simulink model "Tous_le_systeme_2020"  (R2020b)
settings: Solver=FixedStepAuto  StartTime=0.0  StopTime=0.3  FixedStep=1e-6  RelTol=1e-3
undefined symbols (not defined in the file or in its folder): FC, FuelCellLoadFcn, gcbh, ln, sps_rtmsupport, Ts
libraries: simulink x14, powerlib x13, powerlib_meascontrol x3, powerlib_extras x2, pid_lib x1
settings Model: Creator=Abdelhak_Samir  LastModifiedBy=Abdelhak_Samir
settings SolverCC: ZeroCrossAlgorithm=Adaptive
settings DebuggingCC: IgnoredZcDiagnostic=none  UnconnectedInputMsg=none  UnconnectedOutputMsg=none  UnconnectedLineMsg=none
settings ModelReferenceCC: EnableRefExpFcnMdlSchedulingChecks=off

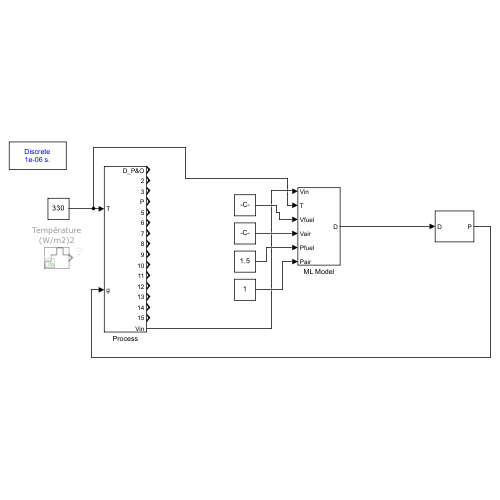
[thumbnail: Simulink's stored preview of the top-level diagram]
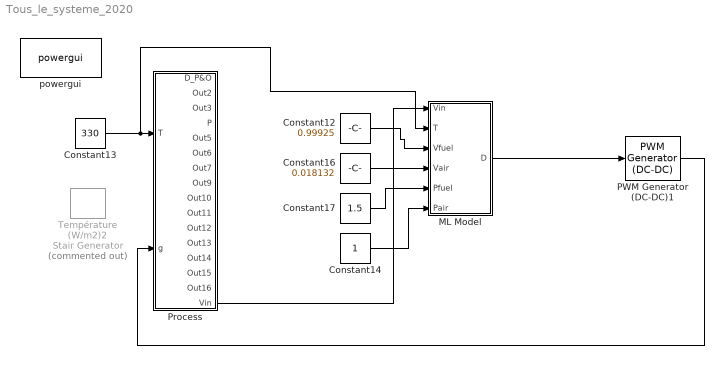
== system Tous_le_systeme_2020 ==
  Constant12 : Constant  Value=0.99925
  Constant13 : Constant  Value=330
  Constant14 : Constant
  Constant16 : Constant  Value=0.018132
  Constant17 : Constant  Value=1.5
  ML Model : Subsystem
  PWM Generator (DC-DC)1 : powerlib_meascontrol/Pulse & Signal Generators/PWM Generator (DC-DC)  Fsw=1/(2e-5)  Ts=1e-6
  Process : Subsystem
  Température (W/m2)2 : powerlib_meascontrol/Pulse & Signal Generators/Stair Generator  Commented=on  t=[0, 0.2 , 0.4 , 0.6, 0.8,1]  e=[300,310,320,330,320,320]  Ts=0.00001
  powergui : powerlib/powergui  Priority=1  SimulationMode=Discrete  SampleTime=1e-6  frequency=60  Iterations=50  frequencyindice=0  Pbase=100e6  ErrMax=1e-4  UnitsV=kV  UnitsW=MW  buscounter=0  FunctionMessages=off  echomessages=off  EnableUseOfTLC=off  CurrentSourceSwitches=off  DisableSnubberDevices=off  DisableRonSwitches=off  DisableVfSwitches=off  DisplayEquations=off  AutomaticDiscreteSolvers=off  SolverType=Tustin/Backward Euler (TBE)  Interpol=off  ExternalGateDelay=off  methode=off  Ts=100  x0status=blocks  SPID=on  SwTol=0  HookPort=off  NonlinearTolerance=1e-4  nMaxIteration=100  ContinueOnMaxIteration=off  RestoreLinks=warning  ResistiveCurrentMeasurement=off  Frange=[0:2:500]  Ylog=off  Xlog=on  ShowGrid=off  save=off  variable=ZData  structure=0  ZoomFFT=off  StartTime=0.0  cycles=1  DisplayStyle=1  fundamental=60  FreqAxis=off  MaxFrequency=1000  frequencyindicesteady=1  RmsSteady=1  display=off
  wires:
  Constant17/1 -> ML Model/5(Pfuel)
  Constant14/1 -> ML Model/6(Pair)
  Constant12/1 -> ML Model/3(Vfuel)
  Constant16/1 -> ML Model/4(Vair)
  Constant13/1 -> ML Model/2(T), Process/1(T)
  Process/16(Vin) -> ML Model/1(Vin)
  ML Model/1(D) -> PWM Generator (DC-DC)1/1
  PWM Generator (DC-DC)1/1 -> Process/2(g)

== system Tous_le_systeme_2020/ML Model ==
  Vin : Inport
  T : Inport  Port=2
  Vfuel : Inport  Port=3
  Vair : Inport  Port=4
  Pfuel : Inport  Port=5
  Pair : Inport  Port=6
  Display : Display
  MATLAB Function1 : MATLAB Function  TreatAsAtomicUnit=on
  MATLAB Function2 : MATLAB Function  Commented=on  TreatAsAtomicUnit=on
  PID Controller : pid_lib/PID Controller  Controller=PID  Form=Parallel  TimeDomain=Discrete-time  UseExternalTs=off  SampleTime=-1  IntegratorMethod=Forward Euler  ControllerParametersSource=internal  P=-150  I=-0.5  D=0.01  N=0  UseFilter=on  TunerSelectOption=Transfer Function Based (PID Tuner App)  InitialConditionSource=internal  InitialConditionForIntegrator=0  InitialConditionForFilter=0  DifferentiatorICPrevScaledInput=0  ExternalReset=none  TrackingMode=off  Kt=1  LimitOutput=off  SatLimitsSource=internal  UpperSaturationLimit=inf  LowerSaturationLimit=-inf  LinearizeAsGain=on  AntiWindupMode=none  Kb=1  POutMin=[]  POutMax=[]  IOutMin=[]  IOutMax=[]  DOutMin=[]  DOutMax=[]  NOutMin=[]  NOutMax=[]  SumOutMin=[]  SumOutMax=[]  SaturationOutMin=[]  SaturationOutMax=[]  PParamMin=[]  PParamMax=[]  IParamMin=[]  IParamMax=[]  DParamMin=[]  DParamMax=[]  NParamMin=[]  NParamMax=[]  KbParamMin=[]  KbParamMax=[]  KtParamMin=[]  KtParamMax=[]  KbOutMin=[]  KbOutMax=[]  KtOutMin=[]  KtOutMax=[]  IntegratorOutMin=[]  IntegratorOutMax=[]  FilterOutMin=[]  FilterOutMax=[]  SumI1OutMin=[]  SumI1OutMax=[]  SumI2OutMin=[]  SumI2OutMax=[]  SumI3OutMin=[]  SumI3OutMax=[]  SumI4OutMin=[]  SumI4OutMax=[]  SumDOutMin=[]  SumDOutMax=[]  DifferentiatorOutMin=[]  DifferentiatorOutMax=[]  FilterDiffOutCoefMin=[]  FilterDiffOutCoefMax=[]  ReciprocalOutMin=[]  ReciprocalOutMax=[]  SumDenOutMin=[]  SumDenOutMax=[]  SumNumOutMin=[]  SumNumOutMax=[]  DivideOutMin=[]  DivideOutMax=[]  UdiffTsProdOutMin=[]  UdiffTsProdOutMax=[]  NTsProdOutMin=[]  NTsProdOutMax=[]  UintegralTsProdOutMin=[]  UintegralTsProdOutMax=[]  UngainTsProdOutMin=[]  UngainTsProdOutMax=[]  IntegratorContinuousStateAttributes=''  IntegratorStateMustResolveToSignalObject=off  IntegratorRTWStateStorageClass=Auto  FilterContinuousStateAttributes=''  FilterStateMustResolveToSignalObject=off  FilterRTWStateStorageClass=Auto  ParallelPVariant=InternalParameters  IdealPVariant=Disabled  IVariant=InternalParameters  DVariant=InternalParameters  IntegratorVariant=Discrete  SatVariant=Disabled  AWVariant=Passthrough  PCopyVariant=Disabled  TRVariant=Disabled  FdbkBlocksVariant=Forward  IdealPFdbkVariant=Disabled  SatFdbkVariant=Disabled  DerivativeFilterVariant=ForwardEulerFilter  NVariant=InternalParameters  NCopyVariant=Disabled  FilterICVariant=InternalICsFilter  IntegratorICVariant=InternalICs  ExternalResetVariant=Disabled  TRSumVariant=Passthrough  SumFdbkVariant=Disabled  SumVariant=Sum_PID  TsampFilterVariant=InternalTs  TsampNgainVariant=Passthrough  TsampIntegralVariant=Disabled_SignalSpec  ExternalSaturationOutDataTypeStr=Inherit: Same as second input
  Saturation1 : Saturate  UpperLimit=0.9  LowerLimit=0.1
  Sum2 : Sum  Inputs=|+-
  D : Outport
  wires:
  Vair/1 -> MATLAB Function1/5(Vair)
  Pfuel/1 -> MATLAB Function1/2(Pfuel)
  T/1 -> MATLAB Function1/1(T)
  Vfuel/1 -> MATLAB Function1/4(Vfuel)
  Pair/1 -> MATLAB Function1/3(Pair)
  Sum2/1 -> PID Controller/1  "Vref-Vin"
  PID Controller/1 -> Saturation1/1
  Vin/1 -> Sum2/2
  Saturation1/1 -> D/1
  MATLAB Function1/1(vmpp) -> Sum2/1, Display/1  "Vref"

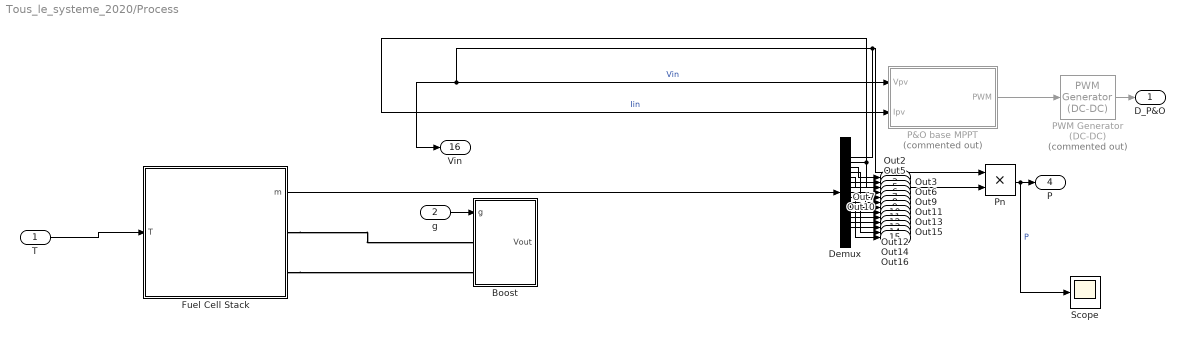
== system Tous_le_systeme_2020/Process ==
  T : Inport
  g : Inport  Port=2
  Boost : Subsystem
  Demux : Demux  Outputs=15
      settings: DisplayOption=none
  Fuel Cell Stack : Subsystem  AncestorBlock=sps_lib/Sources/Fuel Cell Stack  DialogController=POWERSYS.PowerSysDialog  LoadFcn=sps_rtmsupport('LoadFcn',gcbh);FuelCellLoadFcn(gcb)  StartFcn=sps_rtmsupport('StartFcn',gcbh);  StopFcn=sps_rtmsupport('StopFcn',gcbh);  mask(Fuel Cell Stack){PresetModel=PEMFC - 1.26 kW - 24 Vdc, FcType=0, Detailed=Detailed, Eoc=[42,35], NomVI=[52,24.23], EndVI=[100,20], Nc=42, n=46, TOp=55, AirFr=2400, SuppPress=[1.5,1], Comp=[99.95,21,1], SignX=off, SignY=off, FlowRateH2=off, FlowRateAir=off, SystemTemp=on, SystemPH2=off, SystemPAir=off, FCDyn=off, FC_tau=1e-6, Peak_O2=80, V_Under=10}
      mask prompts: PresetModel "Preset model:"; FcType "Fuel Cell type:"; Detailed "Model detail Level:"; Eoc "Voltage at 0A and 1A [V_0(V), V_1(V)]"; NomVI "Nominal operating point [Inom(A), Vnom(V)]"; EndVI "Maximum operating point [Iend(A), Vend(V)]"; Nc "Number of cells"; n "Nominal stack efficiency (%)"; TOp "Operating temperature (Celsius)"; AirFr "Nominal Air flow rate (lpm)"; SuppPress "Nominal supply pressure [Fuel (bar), Air (bar)]"; Comp "Nominal composition (%) [H2 O2 H2O(Air)]"; SignX "Fuel  composition [x_H2(%)]"; SignY "Oxidant composition [y_O2(%)]"; FlowRateH2 "Fuel flow rate [FuelFr(lpm)]"; FlowRateAir "Air flow rate [AirFr(lpm)]"; SystemTemp "System Temperature [T(Kelvin)]"; SystemPH2 "Fuel supply pressure [Pfuel(bar)]"; SystemPAir "Air supply pressure [PAir(bar)]"; FCDyn "Specify Fuel Cell Dynamics?"; FC_tau "Fuel Cell response time (sec)"; Peak_O2 "Peak O2 utilization (%)"; V_Under "Voltage undershoot (V) @ peak O2 utilization"
      mask help:
      | Implements a generic hydrogen fuel cell model which allows the simulation for the following types of cells:
      | - Proton Exchange Membrane Fuel Cell (PEMFC)
      | - Solid Oxide Fuel Cell (SOFC)
      | - Alkaline Fuel Cell (AFC)
      mask init:
      | block = gcb;
      | %% DO NOT CHANGE THIS ORDER
      | FuelCellCback(block,'Inputs')
      | [FC, WantBlockChoice, Ts] = FuelCellInit(block,Eoc,NomVI,EndVI,Nc,n,TOp,AirFr,SuppPress,Comp,FlowRateH2,FlowRateAir);
      | powericon('SetInternalModels','set',block,WantBlockChoice);
      settings: CopyFcn=sps_rtmsupport('CopyFcn',gcbh);  DeleteFcn=sps_rtmsupport('DeleteFcn',gcbh);  UndoDeleteFcn=sps_rtmsupport('UndoDeleteFcn',gcbh);  ModelCloseFcn=sps_rtmsupport('ModelCloseFcn',gcbh);  PreSaveFcn=sps_rtmsupport('PreSaveFcn',gcbh);  PostSaveFcn=sps_rtmsupport('PostSaveFcn',gcbh);  NameChangeFcn=sps_rtmsupport('NameChangeFcn',gcbh);  PreCopyFcn=sps_rtmsupport('PreCopyFcn',gcbh);  OpenFcn=sps_rtmsupport('OpenFcn',gcbh, [1 2 3 13 14 15 16 17 18 19 20]);  CloseFcn=sps_rtmsupport('CloseFcn',gcbh);  PreDeleteFcn=sps_rtmsupport('PreDeleteFcn',gcbh);
      mask Help: helpview(psbhelp)
      mask TypeOptions PresetModel: No (User-Defined) | PEMFC - 1.26 kW - 24 Vdc | PEMFC - 6 kW - 45 Vdc | PEMFC - 50 kW - 625 Vdc | AFC - 2.4 kW - 48 Vdc | SOFC - 3 kW - 100 Vdc | SOFC - 25 kW - 630 Vdc
      mask Callback PresetModel: FuelCellCback(gcb,'Preset')
      mask TypeOptions Detailed: Simplified | Detailed
      mask Callback Detailed: FuelCellCback(gcb,'Visibilities')
      mask Callback FlowRateAir: FuelCellCback(gcb,'Visibilities')
      mask Callback FCDyn: FuelCellCback(gcb,'Visibilities')
      mask DialogControl ParameterTabVar0 Prompt: Parameters
      mask DialogControl plot_graph Prompt: Plot V_I characteristic
      mask DialogControl plot_graph Callback: FuelCellCback(gcb,'PlotGraph');
      mask DialogControl ViewParam Prompt: View Cell parameters
      mask DialogControl ViewParam Callback: FuelCellCback(gcb,'ViewParam');
      mask DialogControl ParameterTabVar01 Prompt: Signal variation
      mask DialogControl ParameterTabVar012 Prompt: Fuel Cell Dynamics
  P&O base MPPT : Subsystem  Commented=on
  PWM Generator (DC-DC) : powerlib_meascontrol/Pulse & Signal Generators/PWM Generator (DC-DC)  Commented=on  Fsw=1/(2e-5)  Ts=1e-6
  Pn : Product
  Scope : Scope
  D_P&O : Outport
  Out2 : Outport  Port=2
  Out3 : Outport  Port=3
  P : Outport  Port=4
  Out5 : Outport  Port=5
  Out6 : Outport  Port=6
  Out7 : Outport  Port=7
  Out9 : Outport  Port=8
  Out10 : Outport  Port=9
  Out11 : Outport  Port=10
  Out12 : Outport  Port=11
  Out13 : Outport  Port=12
  Out14 : Outport  Port=13
  Out15 : Outport  Port=14
  Out16 : Outport  Port=15
  Vin : Outport  Port=16
  wires:
  PWM Generator (DC-DC)/1 -> D_P&O/1
  P&O base MPPT/1(PWM) -> PWM Generator (DC-DC)/1
  Demux/3 -> Out2/1
  Demux/12 -> Out13/1
  Demux/15 -> Out16/1
  Demux/11 -> Out12/1
  Fuel Cell Stack/1(m) -> Demux/1
  Demux/14 -> Out15/1
  Demux/1 -> Vin/1, P&O base MPPT/1(Vpv), Pn/1  "Vin"
  Demux/5 -> Out5/1
  Demux/2 -> Pn/2, P&O base MPPT/2(Ipv)  "Iin"
  T/1 -> Fuel Cell Stack/1(T)
  Demux/4 -> Out3/1
  Demux/9 -> Out10/1
  Demux/7 -> Out7/1
  Demux/6 -> Out6/1
  Demux/8 -> Out9/1
  Demux/10 -> Out11/1
  Demux/13 -> Out14/1
  Pn/1 -> Scope/1, P/1  "P"
  g/1 -> Boost/1(g)
  connections:
  Fuel Cell Stack/RConn1 -- Boost/LConn1
  Fuel Cell Stack/RConn2 -- Boost/LConn2

== system Tous_le_systeme_2020/Process/Boost ==
  note: Voltage Sensor
  note: Boost Convertor
  note: LOAD
  g : Inport
  Current Measurement : powerlib/Measurements/Current Measurement  PhasorSimulation=off  OutputType=Complex  PSBequivalent=0
  Diode : powerlib/Power Electronics/Diode  Ron=0.001  Lon=0  Vf=0.7  IC=0  UseSnubber=0  Rs=500  Cs=250e-9  Measurements=off
  Diode1 : powerlib/Power Electronics/Diode  Ron=0.001  Lon=0  Vf=0.7  IC=0  UseSnubber=0  Rs=500  Cs=250e-9  Measurements=off
  Divide : Product  Inputs=*/
  E1 : Product  Inputs=**
  Mosfet : powerlib/Power Electronics/Mosfet  Ron=0.1  Lon=0  Rd=0.01  Vfd=0.7  IC=0  Rs=1e5  Cs=10^-9  Measurements=off
  Scope : Scope  NumInputPorts=2
  Series RLC Branch : powerlib/Elements/Series RLC Branch  LConnTagsString=__new0  RConnTagsString=__new0  BranchType=L  Resistance=1  Inductance=1e-4  SetiL0=off  InitialCurrent=0  Capacitance=1e-6  Setx0=off  InitialVoltage=0  Measurements=None
  Series RLC Branch1 : powerlib/Elements/Series RLC Branch  LConnTagsString=__new0  RConnTagsString=__new0  BranchType=C  Resistance=1  Inductance=1e-4  SetiL0=off  InitialCurrent=0  Capacitance=4700e-6  Setx0=off  InitialVoltage=0  Measurements=None
  Series RLC Branch4 : powerlib/Elements/Series RLC Branch  LConnTagsString=__new0  RConnTagsString=__new0  BranchType=C  Resistance=1  Inductance=1e-4  SetiL0=off  InitialCurrent=0  Capacitance=4700e-5  Setx0=on  InitialVoltage=42  Measurements=None
  Series RLC Load1 : powerlib/Elements/Series RLC Load  LConnTagsString=a  RConnTagsString=__new0  NominalVoltage=50  NominalFrequency=500  ActivePower=33  InductivePower=0  CapacitivePower=0  Setx0=off  InitialVoltage=0  SetiL0=off  InitialCurrent=0  Measurements=None  LoadType=constant Z
  Voltage Measurement1 : powerlib/Measurements/Voltage Measurement  PhasorSimulation=off  OutputType=Complex  PSBequivalent=0
  a : PMIOPort  Side=Left
  Conn2 : PMIOPort  Port=2  Side=Left
  Vout : Outport
  wires:
  E1/1 -> Scope/1  "Pout"
  Voltage Measurement1/1 -> Vout/1, Divide/1, E1/2  "Vout"
  Current Measurement/1 -> Divide/2, E1/1  "Iout"
  g/1 -> Mosfet/1
  Divide/1 -> ?  "R"
  connections:
  Current Measurement/LConn1 -- Series RLC Branch1/LConn1 -- Diode/RConn1
  Voltage Measurement1/LConn2 -- Series RLC Branch1/RConn1 -- Series RLC Branch4/RConn1 -- Conn2/RConn1 -- Mosfet/RConn1 -- Series RLC Load1/RConn1
  Series RLC Load1/LConn1 -- Current Measurement/RConn1 -- Voltage Measurement1/LConn1
  a/RConn1 -- Diode1/LConn1
  Series RLC Branch/RConn1 -- Mosfet/LConn1 -- Diode/LConn1
  Diode1/RConn1 -- Series RLC Branch4/LConn1 -- Series RLC Branch/LConn1

== system Tous_le_systeme_2020/Process/Fuel Cell Stack ==
  T : Inport
  AirFr : Constant  Value=FC.Uf_O2
  Controlled Voltage Source1 : powerlib/Electrical Sources/Controlled Voltage Source  Initialize=on  Source_Type=AC  Amplitude=0  Phase=0  Frequency=0  Measurements=None
  Current Measurement1 : powerlib/Measurements/Current Measurement  PhasorSimulation=off  OutputType=Complex  PSBequivalent=0
  Diode1 : powerlib/Power Electronics/Diode  Ron=FC.Rohm  Lon=0  Vf=0  IC=0  UseSnubber=off  Rs=1e4  Cs=inf  Measurements=off
  FuelFr : Constant  Value=FC.Uf_H2
  Gain1 : Gain  Gain=0.01
  Gain3 : Gain  Gain=0.01
  Model : Subsystem  AncestorBlock=sps_lib/Sources/Fuel Cell Stack/Model  Variant=on  VariantControlMode=label  LabelModeActiveChoice=Discrete/Detailed
      settings: AttributesFormatString=%<BlockChoice>
  PAir : Constant  Value=FC.PAir
  Pfuel : Constant  Value=FC.Pf
  x_H2 : Constant  Value=FC.x*100
  y_O2 : Constant  Value=FC.y*100
  + : PMIOPort  Tag=PMCPort  Side=Right
  - : PMIOPort  Tag=PMCPort  Port=2  Side=Right
  m : Outport  VectorParamsAs1DForOutWhenUnconnected=off
  wires:
  PAir/1 -> Model/8(PAir)
  Pfuel/1 -> Model/7(Pf)
  T/1 -> Model/2(Op Temp)
  Model/1(Voltage) -> Controlled Voltage Source1/1
  Current Measurement1/1 -> Model/1(Current)
  Model/2(m) -> m/1
  FuelFr/1 -> Model/3(H2)
  x_H2/1 -> Gain1/1
  AirFr/1 -> Model/5(Air)
  y_O2/1 -> Gain3/1
  Gain1/1 -> Model/4(x_H2)
  Gain3/1 -> Model/6(y_O2)
  connections:
  Current Measurement1/LConn1 -- Controlled Voltage Source1/RConn1
  Current Measurement1/RConn1 -- Diode1/LConn1
  -/RConn1 -- Controlled Voltage Source1/LConn1
  Diode1/RConn1 -- +/RConn1

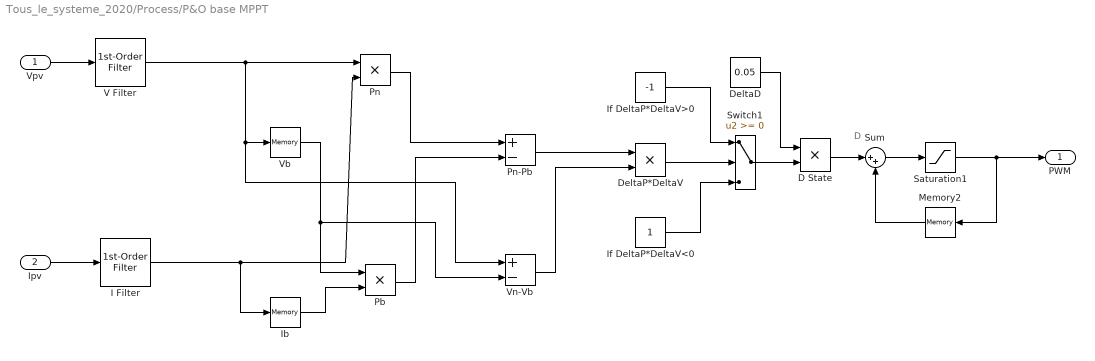
== system Tous_le_systeme_2020/Process/P&O base MPPT ==
  note: D
  Vpv : Inport
  Ipv : Inport  Port=2
  D State : Product  RndMeth=Zero
  DeltaD : Constant  Value=0.05
  DeltaP*DeltaV : Product  RndMeth=Zero
  I Filter : powerlib_extras/Control  Blocks/1st-Order  Filter  FilterType=Lowpass  Tc=1e-3  Initialize=off  Vac_Init=[0.8 -25 60]  Vdc_Init=-0.4  PlotResponse=off  param1=[1 500 1]
  Ib : Memory  InheritSampleTime=on  LinearizeAsDelay=on
  If DeltaP*DeltaV<0 : Constant
  If DeltaP*DeltaV>0 : Constant  Value=-1
  Memory2 : Memory  InheritSampleTime=on
  Pb : Product  RndMeth=Zero
  Pn : Product  RndMeth=Zero
  Pn-Pb : Sum  Inputs=+-
  Saturation1 : Saturate  UpperLimit=0.9  LowerLimit=0.1
  Sum : Sum  Inputs=|++
  Switch1 : Switch
  V Filter : powerlib_extras/Control  Blocks/1st-Order  Filter  FilterType=Lowpass  Tc=1e-3  Initialize=off  Vac_Init=[0.8 -25 60]  Vdc_Init=-0.4  PlotResponse=off  param1=[1 500 1]
  Vb : Memory  InheritSampleTime=on  LinearizeAsDelay=on
  Vn-Vb : Sum  Inputs=+-
  PWM : Outport
  wires:
  Ipv/1 -> I Filter/1
  If DeltaP*DeltaV<0/1 -> Switch1/3
  Pn/1 -> Pn-Pb/1
  V Filter/1 -> Vn-Vb/1, Vb/1, Pn/1
  Ib/1 -> Pb/2
  DeltaP*DeltaV/1 -> Switch1/2
  Vb/1 -> Vn-Vb/2, Pb/1
  If DeltaP*DeltaV>0/1 -> Switch1/1
  Pn-Pb/1 -> DeltaP*DeltaV/1
  Vn-Vb/1 -> DeltaP*DeltaV/2
  I Filter/1 -> Pn/2, Ib/1
  Vpv/1 -> V Filter/1
  Pb/1 -> Pn-Pb/2
  Switch1/1 -> D State/2
  DeltaD/1 -> D State/1
  D State/1 -> Sum/1
  Sum/1 -> Saturation1/1
  Memory2/1 -> Sum/2
  Saturation1/1 -> PWM/1, Memory2/1

== system Tous_le_systeme_2020/Process/Fuel Cell Stack/Model ==
  Current : Inport
  Op Temp : Inport  Port=2
  H2 : Inport  Port=3
  x_H2 : Inport  Port=4
  Air : Inport  Port=5
  y_O2 : Inport  Port=6
  Pf : Inport  Port=7
  PAir : Inport  Port=8
  Continuous/Detailed : Subsystem  VariantControl=Continuous/Detailed
  Continuous/Simplified : Subsystem  VariantControl=Continuous/Simplified
  Discrete/Detailed : Subsystem  VariantControl=Discrete/Detailed
  Discrete/Simplified : Subsystem  VariantControl=Discrete/Simplified
  Voltage : Outport  VectorParamsAs1DForOutWhenUnconnected=off
  m : Outport  Port=2  VectorParamsAs1DForOutWhenUnconnected=off

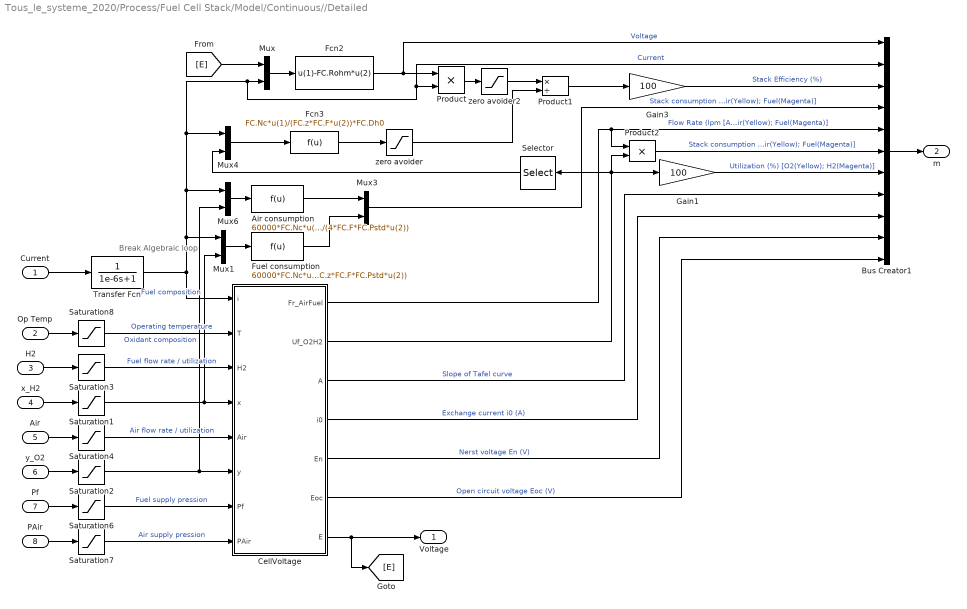
== system Tous_le_systeme_2020/Process/Fuel Cell Stack/Model/Continuous//Detailed ==
  note: Break Algebraic
      | loop
  Current : Inport
  Op Temp : Inport  Port=2
  H2 : Inport  Port=3
  x_H2 : Inport  Port=4
  Air : Inport  Port=5
  y_O2 : Inport  Port=6
  Pf : Inport  Port=7
  PAir : Inport  Port=8
  Air consumption : Fcn  Expr=60000*FC.Nc*u(1)*FC.R*FC.Tstd/(4*FC.F*FC.Pstd*u(2))
  Bus Creator1 : BusCreator  Inputs=11
  CellVoltage : Subsystem
  Fcn2 : Fcn  Expr=u(1)-FC.Rohm*u(2)
  Fcn3 : Fcn  Expr=FC.Nc*u(1)/(FC.z*FC.F*u(2))*FC.Dh0
  Fuel consumption : Fcn  Expr=60000*FC.Nc*u(1)*FC.R*FC.Tstd/(FC.z*FC.F*FC.Pstd*u(2))
  Gain1 : Gain  Gain=100
  Gain3 : Gain  Gain=100
  Mux{,1,3..4,6} (5 alike) : Mux  Inputs=2
  Product : Product  RndMeth=Zero
  Product1 : Product  Inputs=*/  RndMeth=Zero
  Product2 : Product  RndMeth=Zero
  Saturation1 : Saturate  UpperLimit=0.9999  LowerLimit=0.0001
  Saturation2 : Saturate  UpperLimit=0.9999  LowerLimit=0.0001
  Saturation3 : Saturate  UpperLimit=inf  LowerLimit=1e-6
  Saturation4 : Saturate  UpperLimit=inf  LowerLimit=1e-3
  Saturation6 : Saturate  UpperLimit=inf  LowerLimit=0.001
  Saturation7 : Saturate  UpperLimit=inf  LowerLimit=0.001
  Saturation8 : Saturate  UpperLimit=inf  LowerLimit=200
  Selector : Selector  InputPortWidth=2  IndexOptions=Index vector (dialog)  Indices=[2]  OutputSizes=1
  Transfer Fcn : TransferFcn  Denominator=[1e-6 1]
  zero avoider : Saturate  UpperLimit=inf  LowerLimit=1e-6  LinearizeAsGain=off
  zero avoider2 : Saturate  UpperLimit=inf  LowerLimit=0  LinearizeAsGain=off
  Voltage : Outport  VectorParamsAs1DForOutWhenUnconnected=off
  m : Outport  Port=2  VectorParamsAs1DForOutWhenUnconnected=off
  wires:
  [E] -> Mux/1
  CellVoltage/7(E) -> [E], Voltage/1
  CellVoltage/5(En) -> Bus Creator1/10  "Nerst voltage En (V)"
  Saturation2/1 -> Mux6/2, CellVoltage/6(y)  "Oxidant composition"
  CellVoltage/4(i0) -> Bus Creator1/9  "Exchange current i0 (A)"
  Product2/1 -> Bus Creator1/6  "Stack consumption (lpm) [Air(Yellow); Fuel(Magenta)]"
  Gain3/1 -> Bus Creator1/3  "Stack Efficiency (%)"
  CellVoltage/1(Fr_AirFuel) -> Bus Creator1/5, Product2/1  "Flow Rate (lpm [Air(Yellow); Fuel(Magenta)]"
  Fuel consumption/1 -> Mux3/2
  Air consumption/1 -> Mux3/1
  Gain1/1 -> Bus Creator1/7  "Utilization (%) [O2(Yellow); H2(Magenta)]"
  Selector/1 -> Mux4/2
  Mux3/1 -> Bus Creator1/4  "Stack consumption (Standard lpm) [Air(Yellow); Fuel(Magenta)]"
  Saturation4/1 -> CellVoltage/5(Air)  "Air flow rate / utilization"
  Saturation3/1 -> CellVoltage/3(H2)  "Fuel flow rate / utilization"
  Bus Creator1/1 -> m/1
  Mux6/1 -> Air consumption/1
  Mux1/1 -> Fuel consumption/1
  CellVoltage/2(Uf_O2H2) -> Product2/2, Gain1/1, Selector/1
  Transfer Fcn/1 -> Mux6/1, Mux4/1, Mux/2, Bus Creator1/2, Product/2, Mux1/1, CellVoltage/1(i)  "Current"
  Saturation8/1 -> CellVoltage/2(T)  "Operating temperature"
  Saturation7/1 -> CellVoltage/8(PAir)  "Air supply pression"
  Saturation6/1 -> CellVoltage/7(Pf)  "Fuel supply pression"
  Saturation1/1 -> Mux1/2, CellVoltage/4(x)  "Fuel composition"
  Mux4/1 -> Fcn3/1
  PAir/1 -> Saturation7/1
  Pf/1 -> Saturation6/1
  zero avoider2/1 -> Product1/1
  CellVoltage/6(Eoc) -> Bus Creator1/11  "Open circuit voltage Eoc (V)"
  CellVoltage/3(A) -> Bus Creator1/8  "Slope of Tafel curve"
  Air/1 -> Saturation4/1
  Mux/1 -> Fcn2/1
  Fcn2/1 -> Bus Creator1/1, Product/1  "Voltage"
  H2/1 -> Saturation3/1
  x_H2/1 -> Saturation1/1
  y_O2/1 -> Saturation2/1
  Op Temp/1 -> Saturation8/1
  Product/1 -> zero avoider2/1
  Fcn3/1 -> zero avoider/1
  Current/1 -> Transfer Fcn/1
  Product1/1 -> Gain3/1
  zero avoider/1 -> Product1/2

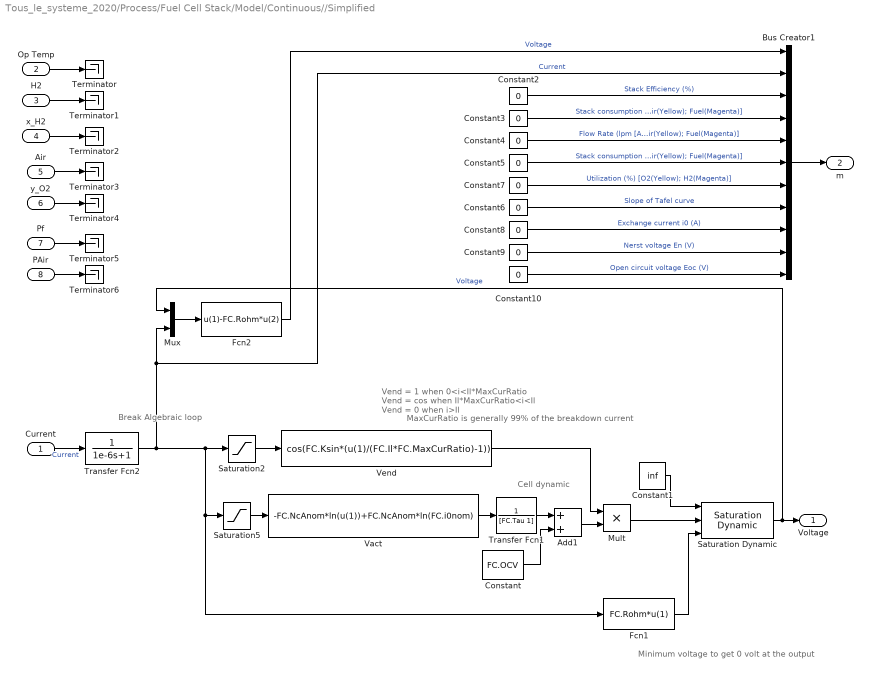
== system Tous_le_systeme_2020/Process/Fuel Cell Stack/Model/Continuous//Simplified ==
  note: MaxCurRatio is generally 99% of the breakdown current
  note: Minimum voltage to get 0 volt at the output
  note: Cell dynamic
  note: Vend = 1 when 0<i<Il*MaxCurRatio
      | Vend = cos when Il*MaxCurRatio<i<Il
      | Vend = 0 when i>Il
  note: Break Algebraic
      | loop
  Current : Inport
  Op Temp : Inport  Port=2
  H2 : Inport  Port=3
  x_H2 : Inport  Port=4
  Air : Inport  Port=5
  y_O2 : Inport  Port=6
  Pf : Inport  Port=7
  PAir : Inport  Port=8
  Add1 : Sum
  Bus Creator1 : BusCreator  Inputs=11
  Constant : Constant  Value=FC.OCV
  Constant1 : Constant  Value=inf
  Constant{2..10} (9 alike) : Constant  Value=0
  Fcn1 : Fcn  Expr=FC.Rohm*u(1)
  Fcn2 : Fcn  Expr=u(1)-FC.Rohm*u(2)
  Mult : Product
  Mux : Mux  Inputs=2
  Saturation Dynamic : simulink/Discontinuities/Saturation Dynamic  OutMin=[]  OutMax=[]  OutDataTypeStr=Inherit: Same as second input  OutDataType=fixdt(1, 16)  OutScaling=2^-10  DoSatur=off
  Saturation2 : Saturate  UpperLimit=FC.Il  LowerLimit=FC.Il*FC.MaxCurRatio  LinearizeAsGain=off
  Saturation5 : Saturate  UpperLimit=inf  LowerLimit=FC.i0nom  LinearizeAsGain=off
  Terminator{,1..6} (7 alike) : Terminator
  Transfer Fcn1 : TransferFcn  Denominator=[FC.Tau 1]
  Transfer Fcn2 : TransferFcn  Denominator=[1e-6 1]
  Vact : Fcn  Expr=-FC.NcAnom*ln(u(1))+FC.NcAnom*ln(FC.i0nom)
  Vend : Fcn  Expr=cos(FC.Ksin*(u(1)/(FC.Il*FC.MaxCurRatio)-1))
  Voltage : Outport  VectorParamsAs1DForOutWhenUnconnected=off
  m : Outport  Port=2  VectorParamsAs1DForOutWhenUnconnected=off
  wires:
  Constant9/1 -> Bus Creator1/10  "Nerst voltage En (V)"
  Constant8/1 -> Bus Creator1/9  "Exchange current i0 (A)"
  Constant5/1 -> Bus Creator1/6  "Stack consumption (lpm) [Air(Yellow); Fuel(Magenta)]"
  Constant2/1 -> Bus Creator1/3  "Stack Efficiency (%)"
  Constant4/1 -> Bus Creator1/5  "Flow Rate (lpm [Air(Yellow); Fuel(Magenta)]"
  Constant7/1 -> Bus Creator1/7  "Utilization (%) [O2(Yellow); H2(Magenta)]"
  Constant3/1 -> Bus Creator1/4  "Stack consumption (Standard lpm) [Air(Yellow); Fuel(Magenta)]"
  Bus Creator1/1 -> m/1
  Constant10/1 -> Bus Creator1/11  "Open circuit voltage Eoc (V)"
  Constant6/1 -> Bus Creator1/8  "Slope of Tafel curve"
  Fcn2/1 -> Bus Creator1/1  "Voltage"
  PAir/1 -> Terminator6/1
  Pf/1 -> Terminator5/1
  Transfer Fcn2/1 -> Bus Creator1/2, Mux/2, Fcn1/1, Saturation5/1, Saturation2/1  "Current"
  Saturation2/1 -> Vend/1
  Vend/1 -> Mult/1
  Mult/1 -> Saturation Dynamic/2
  Add1/1 -> Mult/2
  Vact/1 -> Transfer Fcn1/1
  Fcn1/1 -> Saturation Dynamic/3
  Constant1/1 -> Saturation Dynamic/1
  Constant/1 -> Add1/2
  Transfer Fcn1/1 -> Add1/1
  Saturation Dynamic/1 -> Mux/1, Voltage/1  "Voltage"
  y_O2/1 -> Terminator4/1
  Air/1 -> Terminator3/1
  x_H2/1 -> Terminator2/1
  H2/1 -> Terminator1/1
  Op Temp/1 -> Terminator/1
  Current/1 -> Transfer Fcn2/1  "Current"
  Saturation5/1 -> Vact/1
  Mux/1 -> Fcn2/1

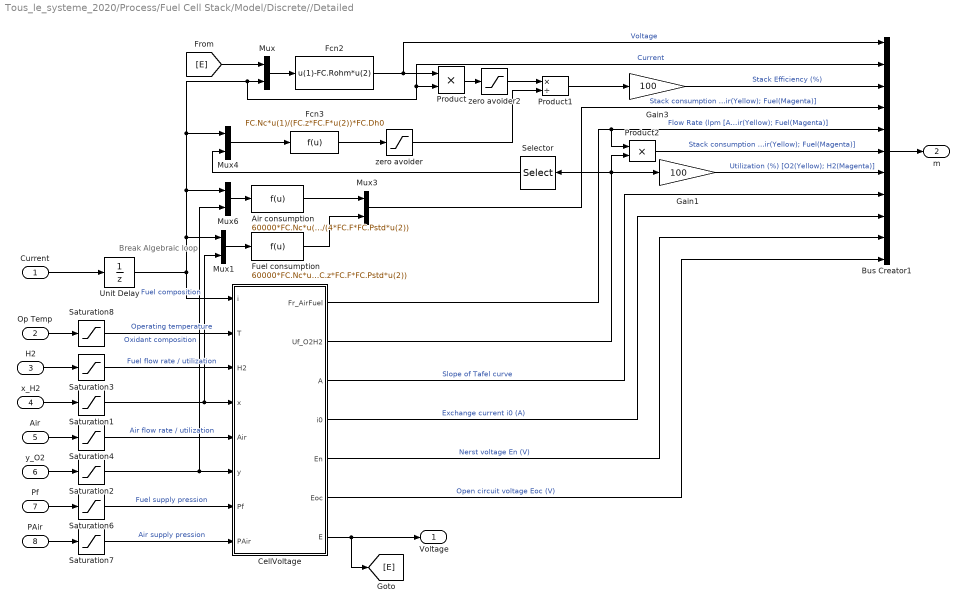
== system Tous_le_systeme_2020/Process/Fuel Cell Stack/Model/Discrete//Detailed ==
  note: Break Algebraic
      | loop
  Current : Inport
  Op Temp : Inport  Port=2
  H2 : Inport  Port=3
  x_H2 : Inport  Port=4
  Air : Inport  Port=5
  y_O2 : Inport  Port=6
  Pf : Inport  Port=7
  PAir : Inport  Port=8
  Air consumption : Fcn  Expr=60000*FC.Nc*u(1)*FC.R*FC.Tstd/(4*FC.F*FC.Pstd*u(2))
  Bus Creator1 : BusCreator  Inputs=11
  CellVoltage : Subsystem
  Fcn2 : Fcn  Expr=u(1)-FC.Rohm*u(2)
  Fcn3 : Fcn  Expr=FC.Nc*u(1)/(FC.z*FC.F*u(2))*FC.Dh0
  Fuel consumption : Fcn  Expr=60000*FC.Nc*u(1)*FC.R*FC.Tstd/(FC.z*FC.F*FC.Pstd*u(2))
  Gain1 : Gain  Gain=100
  Gain3 : Gain  Gain=100
  Mux{,1,3..4,6} (5 alike) : Mux  Inputs=2
  Product : Product  RndMeth=Zero
  Product1 : Product  Inputs=*/  RndMeth=Zero
  Product2 : Product  RndMeth=Zero
  Saturation1 : Saturate  UpperLimit=0.9999  LowerLimit=0.0001
  Saturation2 : Saturate  UpperLimit=0.9999  LowerLimit=0.0001
  Saturation3 : Saturate  UpperLimit=inf  LowerLimit=1e-6
  Saturation4 : Saturate  UpperLimit=inf  LowerLimit=1e-3
  Saturation6 : Saturate  UpperLimit=inf  LowerLimit=0.001
  Saturation7 : Saturate  UpperLimit=inf  LowerLimit=0.001
  Saturation8 : Saturate  UpperLimit=inf  LowerLimit=200
  Selector : Selector  InputPortWidth=2  IndexOptions=Index vector (dialog)  Indices=[2]  OutputSizes=1
  Unit Delay : UnitDelay  SampleTime=Ts  HasFrameUpgradeWarning=on
  zero avoider : Saturate  UpperLimit=inf  LowerLimit=1e-6  LinearizeAsGain=off
  zero avoider2 : Saturate  UpperLimit=inf  LowerLimit=0  LinearizeAsGain=off
  Voltage : Outport  VectorParamsAs1DForOutWhenUnconnected=off
  m : Outport  Port=2  VectorParamsAs1DForOutWhenUnconnected=off
  wires:
  [E] -> Mux/1
  CellVoltage/7(E) -> [E], Voltage/1
  CellVoltage/5(En) -> Bus Creator1/10  "Nerst voltage En (V)"
  Saturation2/1 -> Mux6/2, CellVoltage/6(y)  "Oxidant composition"
  CellVoltage/4(i0) -> Bus Creator1/9  "Exchange current i0 (A)"
  Product2/1 -> Bus Creator1/6  "Stack consumption (lpm) [Air(Yellow); Fuel(Magenta)]"
  Gain3/1 -> Bus Creator1/3  "Stack Efficiency (%)"
  CellVoltage/1(Fr_AirFuel) -> Bus Creator1/5, Product2/1  "Flow Rate (lpm [Air(Yellow); Fuel(Magenta)]"
  Fuel consumption/1 -> Mux3/2
  Air consumption/1 -> Mux3/1
  Gain1/1 -> Bus Creator1/7  "Utilization (%) [O2(Yellow); H2(Magenta)]"
  Selector/1 -> Mux4/2
  Mux3/1 -> Bus Creator1/4  "Stack consumption (Standard lpm) [Air(Yellow); Fuel(Magenta)]"
  Saturation4/1 -> CellVoltage/5(Air)  "Air flow rate / utilization"
  Saturation3/1 -> CellVoltage/3(H2)  "Fuel flow rate / utilization"
  Bus Creator1/1 -> m/1
  Mux6/1 -> Air consumption/1
  Mux1/1 -> Fuel consumption/1
  CellVoltage/2(Uf_O2H2) -> Product2/2, Gain1/1, Selector/1
  Unit Delay/1 -> Mux6/1, Mux4/1, Mux/2, Bus Creator1/2, Product/2, Mux1/1, CellVoltage/1(i)  "Current"
  Saturation8/1 -> CellVoltage/2(T)  "Operating temperature"
  Saturation7/1 -> CellVoltage/8(PAir)  "Air supply pression"
  Saturation6/1 -> CellVoltage/7(Pf)  "Fuel supply pression"
  Saturation1/1 -> Mux1/2, CellVoltage/4(x)  "Fuel composition"
  Mux4/1 -> Fcn3/1
  PAir/1 -> Saturation7/1
  Pf/1 -> Saturation6/1
  zero avoider2/1 -> Product1/1
  CellVoltage/6(Eoc) -> Bus Creator1/11  "Open circuit voltage Eoc (V)"
  CellVoltage/3(A) -> Bus Creator1/8  "Slope of Tafel curve"
  Air/1 -> Saturation4/1
  Mux/1 -> Fcn2/1
  Fcn2/1 -> Bus Creator1/1, Product/1  "Voltage"
  H2/1 -> Saturation3/1
  x_H2/1 -> Saturation1/1
  y_O2/1 -> Saturation2/1
  Op Temp/1 -> Saturation8/1
  Product/1 -> zero avoider2/1
  Fcn3/1 -> zero avoider/1
  Current/1 -> Unit Delay/1
  Product1/1 -> Gain3/1
  zero avoider/1 -> Product1/2

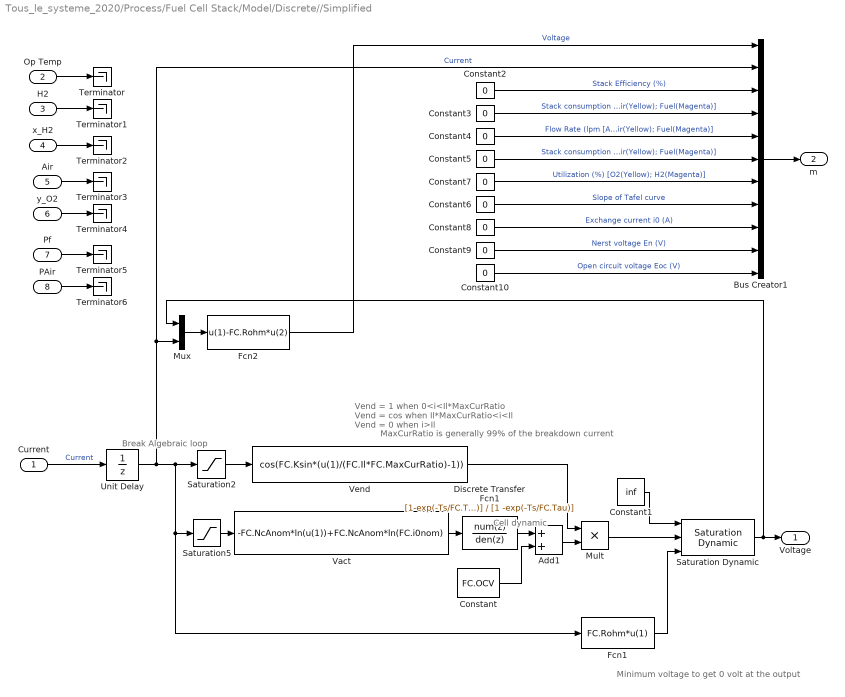
== system Tous_le_systeme_2020/Process/Fuel Cell Stack/Model/Discrete//Simplified ==
  note: MaxCurRatio is generally 99% of the breakdown current
  note: Minimum voltage to get 0 volt at the output
  note: Cell dynamic
  note: Vend = 1 when 0<i<Il*MaxCurRatio
      | Vend = cos when Il*MaxCurRatio<i<Il
      | Vend = 0 when i>Il
  note: Break Algebraic
      | loop
  Current : Inport
  Op Temp : Inport  Port=2
  H2 : Inport  Port=3
  x_H2 : Inport  Port=4
  Air : Inport  Port=5
  y_O2 : Inport  Port=6
  Pf : Inport  Port=7
  PAir : Inport  Port=8
  Add1 : Sum
  Bus Creator1 : BusCreator  Inputs=11
  Constant : Constant  Value=FC.OCV
  Constant1 : Constant  Value=inf
  Constant{2..10} (9 alike) : Constant  Value=0
  Discrete Transfer Fcn1 : DiscreteTransferFcn  Numerator=[1-exp(-Ts/FC.Tau)]  Denominator=[1 -exp(-Ts/FC.Tau)]  SampleTime=Ts
  Fcn1 : Fcn  Expr=FC.Rohm*u(1)
  Fcn2 : Fcn  Expr=u(1)-FC.Rohm*u(2)
  Mult : Product
  Mux : Mux  Inputs=2
  Saturation Dynamic : simulink/Discontinuities/Saturation Dynamic  OutMin=[]  OutMax=[]  OutDataTypeStr=Inherit: Same as second input  OutDataType=fixdt(1, 16)  OutScaling=2^-10  DoSatur=off
  Saturation2 : Saturate  UpperLimit=FC.Il  LowerLimit=FC.Il*FC.MaxCurRatio  LinearizeAsGain=off
  Saturation5 : Saturate  UpperLimit=inf  LowerLimit=FC.i0nom  LinearizeAsGain=off
  Terminator{,1..6} (7 alike) : Terminator
  Unit Delay : UnitDelay  SampleTime=Ts  HasFrameUpgradeWarning=on
  Vact : Fcn  Expr=-FC.NcAnom*ln(u(1))+FC.NcAnom*ln(FC.i0nom)
  Vend : Fcn  Expr=cos(FC.Ksin*(u(1)/(FC.Il*FC.MaxCurRatio)-1))
  Voltage : Outport  VectorParamsAs1DForOutWhenUnconnected=off
  m : Outport  Port=2  VectorParamsAs1DForOutWhenUnconnected=off
  wires:
  Fcn2/1 -> Bus Creator1/1  "Voltage"
  Constant9/1 -> Bus Creator1/10  "Nerst voltage En (V)"
  Constant8/1 -> Bus Creator1/9  "Exchange current i0 (A)"
  Constant5/1 -> Bus Creator1/6  "Stack consumption (lpm) [Air(Yellow); Fuel(Magenta)]"
  Constant2/1 -> Bus Creator1/3  "Stack Efficiency (%)"
  Constant4/1 -> Bus Creator1/5  "Flow Rate (lpm [Air(Yellow); Fuel(Magenta)]"
  Constant7/1 -> Bus Creator1/7  "Utilization (%) [O2(Yellow); H2(Magenta)]"
  Constant3/1 -> Bus Creator1/4  "Stack consumption (Standard lpm) [Air(Yellow); Fuel(Magenta)]"
  Bus Creator1/1 -> m/1
  Constant10/1 -> Bus Creator1/11  "Open circuit voltage Eoc (V)"
  Constant6/1 -> Bus Creator1/8  "Slope of Tafel curve"
  PAir/1 -> Terminator6/1
  Pf/1 -> Terminator5/1
  Unit Delay/1 -> Bus Creator1/2, Mux/2, Fcn1/1, Saturation5/1, Saturation2/1  "Current"
  Saturation2/1 -> Vend/1
  Vend/1 -> Mult/1
  Mult/1 -> Saturation Dynamic/2
  Add1/1 -> Mult/2
  Vact/1 -> Discrete Transfer Fcn1/1
  Fcn1/1 -> Saturation Dynamic/3
  Constant1/1 -> Saturation Dynamic/1
  Constant/1 -> Add1/2
  Discrete Transfer Fcn1/1 -> Add1/1
  Saturation Dynamic/1 -> Mux/1, Voltage/1
  y_O2/1 -> Terminator4/1
  Air/1 -> Terminator3/1
  x_H2/1 -> Terminator2/1
  H2/1 -> Terminator1/1
  Op Temp/1 -> Terminator/1
  Current/1 -> Unit Delay/1  "Current"
  Saturation5/1 -> Vact/1
  Mux/1 -> Fcn2/1

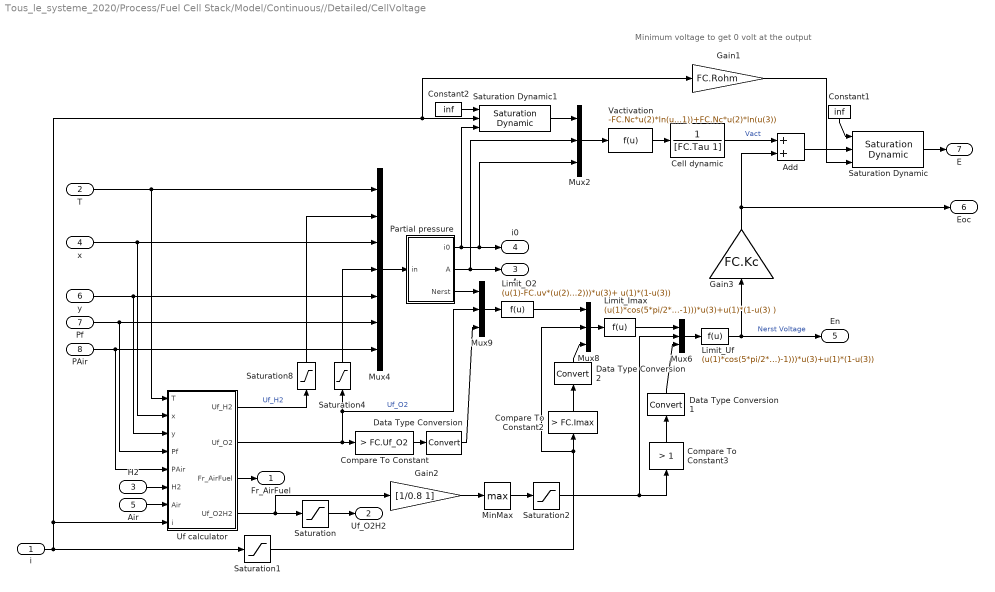
== system Tous_le_systeme_2020/Process/Fuel Cell Stack/Model/Continuous//Detailed/CellVoltage ==
  note: Minimum voltage to get 0 volt at the output
  i : Inport
  T : Inport  Port=2
  H2 : Inport  Port=3
  x : Inport  Port=4
  Air : Inport  Port=5
  y : Inport  Port=6
  Pf : Inport  Port=7
  PAir : Inport  Port=8
  Add : Sum
  Cell dynamic : TransferFcn  Denominator=[FC.Tau 1]
  Compare To Constant : simulink/Logic and Bit Operations/Compare To Constant  relop=>  const=FC.Uf_O2  OutDataTypeStr=boolean
  Compare To Constant2 : simulink/Logic and Bit Operations/Compare To Constant  relop=>  const=FC.Imax  OutDataTypeStr=boolean
  Compare To Constant3 : simulink/Logic and Bit Operations/Compare To Constant  relop=>  const=1  OutDataTypeStr=boolean
  Constant1 : Constant  Value=inf
  Constant2 : Constant  Value=inf
  Data Type Conversion : DataTypeConversion
  Data Type Conversion1 : DataTypeConversion
  Data Type Conversion2 : DataTypeConversion
  Gain1 : Gain  Gain=FC.Rohm
  Gain2 : Gain  Gain=[1/0.8 1]
  Gain3 : Gain  Gain=FC.Kc
  Limit_Imax : Fcn  Expr=(u(1)*cos(5*pi/2*(u(2)/FC.Imax-1)))*u(3)+u(1)*(1-u(3) )
  Limit_O2 : Fcn  Expr=(u(1)-FC.uv*(u(2)-FC.Uf_O2)/(FC.Kc*(FC.ufO2max-FC.Uf_O2)))*u(3)+ u(1)*(1-u(3))
  Limit_Uf : Fcn  Expr=(u(1)*cos(5*pi/2*(u(2)-1)))*u(3)+u(1)*(1-u(3))
  MinMax : MinMax  Function=max
  Mux{2,6,8..9} (4 alike) : Mux  Inputs=3
  Mux4 : Mux  Inputs=7
  Partial pressure : Subsystem
  Saturation : Saturate  UpperLimit=0.9999  LowerLimit=0.0001
  Saturation Dynamic : simulink/Discontinuities/Saturation Dynamic  OutMin=[]  OutMax=[]  OutDataTypeStr=Inherit: Same as second input  OutDataType=fixdt(1, 16)  OutScaling=2^-10  DoSatur=off
  Saturation Dynamic1 : simulink/Discontinuities/Saturation Dynamic  OutMin=[]  OutMax=[]  OutDataTypeStr=Inherit: Same as second input  OutDataType=fixdt(1, 16)  OutScaling=2^-10  DoSatur=off
  Saturation1 : Saturate  UpperLimit=FC.Imax*1.2  LowerLimit=0
  Saturation2 : Saturate  UpperLimit=1.2  LowerLimit=0
  Saturation4 : Saturate  UpperLimit=FC.Uf_O2  LowerLimit=0
  Saturation8 : Saturate  UpperLimit=FC.Uf_H2  LowerLimit=0
  Uf calculator : Subsystem
  Vactivation : Fcn  Expr=-FC.Nc*u(2)*ln(u(1))+FC.Nc*u(2)*ln(u(3))
  Fr_AirFuel : Outport  VectorParamsAs1DForOutWhenUnconnected=off
  Uf_O2H2 : Outport  Port=2  VectorParamsAs1DForOutWhenUnconnected=off
  A : Outport  Port=3  VectorParamsAs1DForOutWhenUnconnected=off
  i0 : Outport  Port=4  VectorParamsAs1DForOutWhenUnconnected=off
  En : Outport  Port=5  VectorParamsAs1DForOutWhenUnconnected=off
  Eoc : Outport  Port=6  VectorParamsAs1DForOutWhenUnconnected=off
  E : Outport  Port=7  VectorParamsAs1DForOutWhenUnconnected=off
  wires:
  Gain3/1 -> Eoc/1, Add/2
  Data Type Conversion1/1 -> Mux6/3
  Compare To Constant3/1 -> Data Type Conversion1/1
  Saturation2/1 -> Mux6/2, Compare To Constant3/1
  Saturation1/1 -> Mux8/2, Compare To Constant2/1
  Compare To Constant2/1 -> Data Type Conversion2/1
  Data Type Conversion2/1 -> Mux8/3
  Data Type Conversion/1 -> Mux9/3
  Compare To Constant/1 -> Data Type Conversion/1
  Gain2/1 -> MinMax/1
  Partial pressure/3(Nerst) -> Mux9/1
  Saturation4/1 -> Mux4/4
  MinMax/1 -> Saturation2/1
  Saturation/1 -> Uf_O2H2/1
  Mux6/1 -> Limit_Uf/1
  Gain1/1 -> Saturation Dynamic/3
  Constant1/1 -> Saturation Dynamic/1
  Saturation Dynamic/1 -> E/1
  Add/1 -> Saturation Dynamic/2
  Cell dynamic/1 -> Add/1  "Vact"
  Vactivation/1 -> Cell dynamic/1
  Mux2/1 -> Vactivation/1
  Saturation Dynamic1/1 -> Mux2/1
  Constant2/1 -> Saturation Dynamic1/1
  Mux4/1 -> Partial pressure/1(in)
  Uf calculator/4(Uf_O2H2) -> Gain2/1, Saturation/1
  Saturation8/1 -> Mux4/2
  Limit_O2/1 -> Mux8/1
  Mux9/1 -> Limit_O2/1
  Uf calculator/3(Fr_AirFuel) -> Fr_AirFuel/1
  Limit_Uf/1 -> Gain3/1, En/1  "Nerst Voltage"
  Limit_Imax/1 -> Mux6/1
  Mux8/1 -> Limit_Imax/1
  Air/1 -> Uf calculator/7(Air)
  Uf calculator/2(Uf_O2) -> Mux9/2, Saturation4/1, Compare To Constant/1  "Uf_O2"
  Uf calculator/1(Uf_H2) -> Saturation8/1  "Uf_H2"
  i/1 -> Saturation1/1, Uf calculator/8(i), Gain1/1, Saturation Dynamic1/2
  H2/1 -> Uf calculator/6(H2)
  Partial pressure/2(A) -> Mux2/2, A/1
  Partial pressure/1(i0) -> Mux2/3, i0/1, Saturation Dynamic1/3
  PAir/1 -> Uf calculator/5(PAir), Mux4/7
  Pf/1 -> Uf calculator/4(Pf), Mux4/6
  y/1 -> Uf calculator/3(y), Mux4/5
  x/1 -> Uf calculator/2(x), Mux4/3
  T/1 -> Uf calculator/1(T), Mux4/1

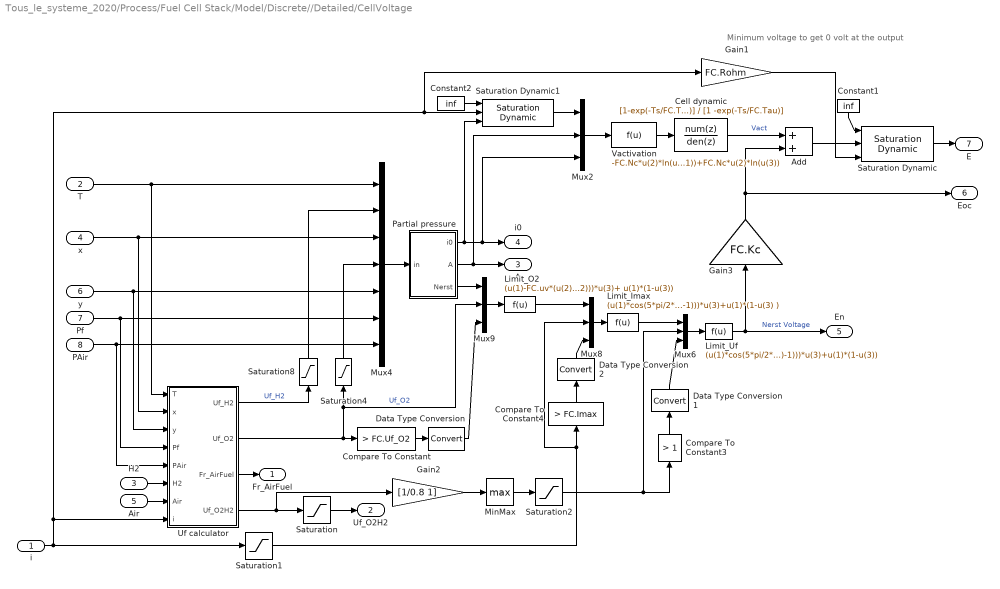
== system Tous_le_systeme_2020/Process/Fuel Cell Stack/Model/Discrete//Detailed/CellVoltage ==
  note: Minimum voltage to get 0 volt at the output
  i : Inport
  T : Inport  Port=2
  H2 : Inport  Port=3
  x : Inport  Port=4
  Air : Inport  Port=5
  y : Inport  Port=6
  Pf : Inport  Port=7
  PAir : Inport  Port=8
  Add : Sum
  Cell dynamic : DiscreteTransferFcn  Numerator=[1-exp(-Ts/FC.Tau)]  Denominator=[1 -exp(-Ts/FC.Tau)]  SampleTime=Ts
  Compare To Constant : simulink/Logic and Bit Operations/Compare To Constant  relop=>  const=FC.Uf_O2  OutDataTypeStr=boolean
  Compare To Constant3 : simulink/Logic and Bit Operations/Compare To Constant  relop=>  const=1  OutDataTypeStr=boolean
  Compare To Constant4 : simulink/Logic and Bit Operations/Compare To Constant  relop=>  const=FC.Imax  OutDataTypeStr=boolean
  Constant1 : Constant  Value=inf
  Constant2 : Constant  Value=inf
  Data Type Conversion : DataTypeConversion
  Data Type Conversion1 : DataTypeConversion
  Data Type Conversion2 : DataTypeConversion
  Gain1 : Gain  Gain=FC.Rohm
  Gain2 : Gain  Gain=[1/0.8 1]
  Gain3 : Gain  Gain=FC.Kc
  Limit_Imax : Fcn  Expr=(u(1)*cos(5*pi/2*(u(2)/FC.Imax-1)))*u(3)+u(1)*(1-u(3) )
  Limit_O2 : Fcn  Expr=(u(1)-FC.uv*(u(2)-FC.Uf_O2)/(FC.Kc*(FC.ufO2max-FC.Uf_O2)))*u(3)+ u(1)*(1-u(3))
  Limit_Uf : Fcn  Expr=(u(1)*cos(5*pi/2*(u(2)-1)))*u(3)+u(1)*(1-u(3))
  MinMax : MinMax  Function=max
  Mux{2,6,8..9} (4 alike) : Mux  Inputs=3
  Mux4 : Mux  Inputs=7
  Partial pressure : Subsystem
  Saturation : Saturate  UpperLimit=0.9999  LowerLimit=0.0001
  Saturation Dynamic : simulink/Discontinuities/Saturation Dynamic  OutMin=[]  OutMax=[]  OutDataTypeStr=Inherit: Same as second input  OutDataType=fixdt(1, 16)  OutScaling=2^-10  DoSatur=off
  Saturation Dynamic1 : simulink/Discontinuities/Saturation Dynamic  OutMin=[]  OutMax=[]  OutDataTypeStr=Inherit: Same as second input  OutDataType=fixdt(1, 16)  OutScaling=2^-10  DoSatur=off
  Saturation1 : Saturate  UpperLimit=FC.Imax*1.2  LowerLimit=0
  Saturation2 : Saturate  UpperLimit=1.2  LowerLimit=0
  Saturation4 : Saturate  UpperLimit=FC.Uf_O2  LowerLimit=0
  Saturation8 : Saturate  UpperLimit=FC.Uf_H2  LowerLimit=0
  Uf calculator : Subsystem
  Vactivation : Fcn  Expr=-FC.Nc*u(2)*ln(u(1))+FC.Nc*u(2)*ln(u(3))
  Fr_AirFuel : Outport  VectorParamsAs1DForOutWhenUnconnected=off
  Uf_O2H2 : Outport  Port=2  VectorParamsAs1DForOutWhenUnconnected=off
  A : Outport  Port=3  VectorParamsAs1DForOutWhenUnconnected=off
  i0 : Outport  Port=4  VectorParamsAs1DForOutWhenUnconnected=off
  En : Outport  Port=5  VectorParamsAs1DForOutWhenUnconnected=off
  Eoc : Outport  Port=6  VectorParamsAs1DForOutWhenUnconnected=off
  E : Outport  Port=7  VectorParamsAs1DForOutWhenUnconnected=off
  wires:
  Gain3/1 -> Eoc/1, Add/2
  T/1 -> Uf calculator/1(T), Mux4/1
  x/1 -> Mux4/3, Uf calculator/2(x)
  y/1 -> Mux4/5, Uf calculator/3(y)
  Pf/1 -> Mux4/6, Uf calculator/4(Pf)
  PAir/1 -> Mux4/7, Uf calculator/5(PAir)
  Partial pressure/1(i0) -> Saturation Dynamic1/3, i0/1, Mux2/3
  Partial pressure/2(A) -> A/1, Mux2/2
  H2/1 -> Uf calculator/6(H2)
  i/1 -> Uf calculator/8(i), Saturation Dynamic1/2, Gain1/1, Saturation1/1
  Uf calculator/1(Uf_H2) -> Saturation8/1  "Uf_H2"
  Uf calculator/2(Uf_O2) -> Compare To Constant/1, Saturation4/1, Mux9/2  "Uf_O2"
  Air/1 -> Uf calculator/7(Air)
  Mux8/1 -> Limit_Imax/1
  Limit_Imax/1 -> Mux6/1
  Limit_Uf/1 -> Gain3/1, En/1  "Nerst Voltage"
  Uf calculator/3(Fr_AirFuel) -> Fr_AirFuel/1
  Mux9/1 -> Limit_O2/1
  Limit_O2/1 -> Mux8/1
  Saturation8/1 -> Mux4/2
  Uf calculator/4(Uf_O2H2) -> Saturation/1, Gain2/1
  Mux4/1 -> Partial pressure/1(in)
  Constant2/1 -> Saturation Dynamic1/1
  Saturation Dynamic1/1 -> Mux2/1
  Mux2/1 -> Vactivation/1
  Vactivation/1 -> Cell dynamic/1
  Cell dynamic/1 -> Add/1  "Vact"
  Add/1 -> Saturation Dynamic/2
  Saturation Dynamic/1 -> E/1
  Constant1/1 -> Saturation Dynamic/1
  Gain1/1 -> Saturation Dynamic/3
  Mux6/1 -> Limit_Uf/1
  Saturation/1 -> Uf_O2H2/1
  MinMax/1 -> Saturation2/1
  Saturation4/1 -> Mux4/4
  Partial pressure/3(Nerst) -> Mux9/1
  Gain2/1 -> MinMax/1
  Compare To Constant/1 -> Data Type Conversion/1
  Data Type Conversion/1 -> Mux9/3
  Data Type Conversion2/1 -> Mux8/3
  Compare To Constant4/1 -> Data Type Conversion2/1
  Saturation1/1 -> Mux8/2, Compare To Constant4/1
  Saturation2/1 -> Mux6/2, Compare To Constant3/1
  Compare To Constant3/1 -> Data Type Conversion1/1
  Data Type Conversion1/1 -> Mux6/3

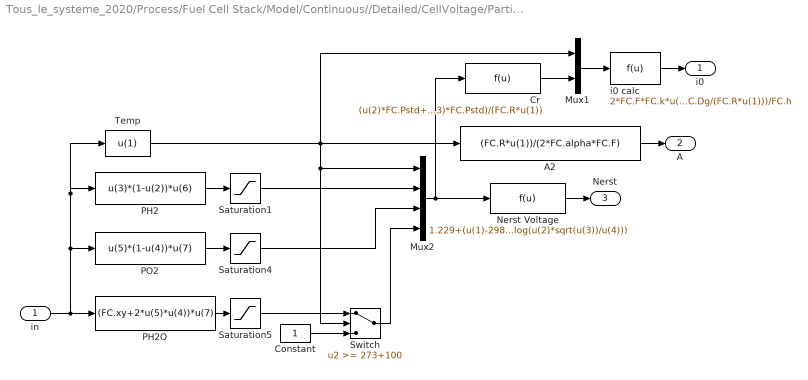
== system Tous_le_systeme_2020/Process/Fuel Cell Stack/Model/Continuous//Detailed/CellVoltage/Partial pressure ==
  in : Inport
  A2 : Fcn  Expr=(FC.R*u(1))/(2*FC.alpha*FC.F)
  Constant : Constant
  Cr : Fcn  Expr=(u(2)*FC.Pstd+u(3)*FC.Pstd)/(FC.R*u(1))
  Mux1 : Mux  Inputs=2
  Mux2 : Mux
  Nerst Voltage : Fcn  Expr=1.229+(u(1)-298.15)*(-44.43/(FC.z*FC.F))+(FC.R*u(1)/(FC.z*FC.F))*(log(u(2)*sqrt(u(3))/u(4)))
  PH2 : Fcn  Expr=u(3)*(1-u(2))*u(6)
  PH2O : Fcn  Expr=(FC.xy+2*u(5)*u(4))*u(7)
  PO2 : Fcn  Expr=u(5)*(1-u(4))*u(7)
  Saturation1 : Saturate  UpperLimit=inf  LowerLimit=0.0001
  Saturation4 : Saturate  UpperLimit=inf  LowerLimit=0.0001
  Saturation5 : Saturate  UpperLimit=inf  LowerLimit=0.0001
  Switch : Switch  Threshold=273+100
  Temp : Fcn  Expr=u(1)
  i0 calc : Fcn  Expr=2*FC.F*FC.k*u(1)*u(2)*exp(-FC.Dg/(FC.R*u(1)))/FC.h
  i0 : Outport  VectorParamsAs1DForOutWhenUnconnected=off
  A : Outport  Port=2  VectorParamsAs1DForOutWhenUnconnected=off
  Nerst : Outport  Port=3  VectorParamsAs1DForOutWhenUnconnected=off
  wires:
  Temp/1 -> Mux2/1, Switch/2, A2/1, Mux1/1
  i0 calc/1 -> i0/1
  Nerst Voltage/1 -> Nerst/1
  A2/1 -> A/1
  PH2O/1 -> Saturation5/1
  PO2/1 -> Saturation4/1
  PH2/1 -> Saturation1/1
  Saturation1/1 -> Mux2/2
  Saturation4/1 -> Mux2/3
  Switch/1 -> Mux2/4
  Saturation5/1 -> Switch/1
  Constant/1 -> Switch/3
  Mux2/1 -> Nerst Voltage/1, Cr/1
  in/1 -> PH2O/1, Temp/1, PH2/1, PO2/1
  Mux1/1 -> i0 calc/1
  Cr/1 -> Mux1/2

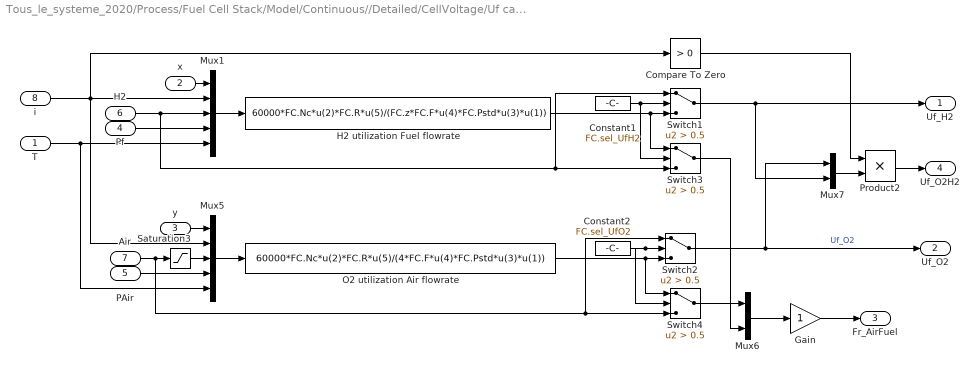
== system Tous_le_systeme_2020/Process/Fuel Cell Stack/Model/Continuous//Detailed/CellVoltage/Uf calculator ==
  T : Inport
  x : Inport  Port=2
  y : Inport  Port=3
  Pf : Inport  Port=4
  PAir : Inport  Port=5
  H2 : Inport  Port=6
  Air : Inport  Port=7
  i : Inport  Port=8
  Compare To Zero : simulink/Logic and Bit Operations/Compare To Zero  relop=>  OutDataTypeStr=uint8
  Constant1 : Constant  Value=FC.sel_UfH2
  Constant2 : Constant  Value=FC.sel_UfO2
  Gain : Gain
  H2 utilization Fuel flowrate : Fcn  Expr=60000*FC.Nc*u(2)*FC.R*u(5)/(FC.z*FC.F*u(4)*FC.Pstd*u(3)*u(1))
  Mux1 : Mux  Inputs=5
  Mux5 : Mux  Inputs=5
  Mux6 : Mux  Inputs=2
  Mux7 : Mux  Inputs=2
  O2 utilization Air flowrate : Fcn  Expr=60000*FC.Nc*u(2)*FC.R*u(5)/(4*FC.F*u(4)*FC.Pstd*u(3)*u(1))
  Product2 : Product  RndMeth=Zero
  Saturation3 : Saturate  UpperLimit=inf  LowerLimit=FC.AirFr_Max*0.01
  Switch{1..4} (4 alike) : Switch  Criteria=u2 > Threshold  Threshold=0.5
  Uf_H2 : Outport  VectorParamsAs1DForOutWhenUnconnected=off
  Uf_O2 : Outport  Port=2  VectorParamsAs1DForOutWhenUnconnected=off
  Fr_AirFuel : Outport  Port=3  VectorParamsAs1DForOutWhenUnconnected=off
  Uf_O2H2 : Outport  Port=4  VectorParamsAs1DForOutWhenUnconnected=off
  wires:
  Switch1/1 -> Mux7/2, Uf_H2/1
  Saturation3/1 -> Mux5/3
  Switch2/1 -> Mux7/1, Uf_O2/1  "Uf_O2"
  Gain/1 -> Fr_AirFuel/1
  Switch4/1 -> Mux6/1
  Switch3/1 -> Mux6/2
  Mux6/1 -> Gain/1
  PAir/1 -> Mux5/4
  Pf/1 -> Mux1/4
  T/1 -> Mux1/5, Mux5/5
  O2 utilization Air flowrate/1 -> Switch4/1, Switch2/3
  Constant2/1 -> Switch4/2, Switch2/2
  Constant1/1 -> Switch3/2, Switch1/2
  H2 utilization Fuel flowrate/1 -> Switch3/1, Switch1/3
  i/1 -> Compare To Zero/1, Mux1/2, Mux5/2
  Air/1 -> Saturation3/1, Switch2/1, Switch4/3
  y/1 -> Mux5/1
  H2/1 -> Mux1/3, Switch1/1, Switch3/3
  x/1 -> Mux1/1
  Mux5/1 -> O2 utilization Air flowrate/1
  Mux1/1 -> H2 utilization Fuel flowrate/1
  Mux7/1 -> Product2/2
  Product2/1 -> Uf_O2H2/1
  Compare To Zero/1 -> Product2/1

== system Tous_le_systeme_2020/Process/Fuel Cell Stack/Model/Discrete//Detailed/CellVoltage/Partial pressure ==
  in : Inport
  A2 : Fcn  Expr=(FC.R*u(1))/(2*FC.alpha*FC.F)
  Constant : Constant
  Cr : Fcn  Expr=(u(2)*FC.Pstd+u(3)*FC.Pstd)/(FC.R*u(1))
  Mux1 : Mux  Inputs=2
  Mux2 : Mux
  Nerst Voltage : Fcn  Expr=1.229+(u(1)-298.15)*(-44.43/(FC.z*FC.F))+(FC.R*u(1)/(FC.z*FC.F))*(log(u(2)*sqrt(u(3))/u(4)))
  PH2 : Fcn  Expr=u(3)*(1-u(2))*u(6)
  PH2O : Fcn  Expr=(FC.xy+2*u(5)*u(4))*u(7)
  PO2 : Fcn  Expr=u(5)*(1-u(4))*u(7)
  Saturation1 : Saturate  UpperLimit=inf  LowerLimit=0.0001
  Saturation4 : Saturate  UpperLimit=inf  LowerLimit=0.0001
  Saturation5 : Saturate  UpperLimit=inf  LowerLimit=0.0001
  Switch : Switch  Threshold=273+100
  Temp : Fcn  Expr=u(1)
  i0 calc : Fcn  Expr=2*FC.F*FC.k*u(1)*u(2)*exp(-FC.Dg/(FC.R*u(1)))/FC.h
  i0 : Outport  VectorParamsAs1DForOutWhenUnconnected=off
  A : Outport  Port=2  VectorParamsAs1DForOutWhenUnconnected=off
  Nerst : Outport  Port=3  VectorParamsAs1DForOutWhenUnconnected=off
  wires:
  Cr/1 -> Mux1/2
  Mux1/1 -> i0 calc/1
  in/1 -> PO2/1, PH2/1, Temp/1, PH2O/1
  Mux2/1 -> Cr/1, Nerst Voltage/1
  Constant/1 -> Switch/3
  Saturation5/1 -> Switch/1
  Switch/1 -> Mux2/4
  Saturation4/1 -> Mux2/3
  Saturation1/1 -> Mux2/2
  PH2/1 -> Saturation1/1
  PO2/1 -> Saturation4/1
  PH2O/1 -> Saturation5/1
  A2/1 -> A/1
  Nerst Voltage/1 -> Nerst/1
  i0 calc/1 -> i0/1
  Temp/1 -> Mux1/1, A2/1, Switch/2, Mux2/1

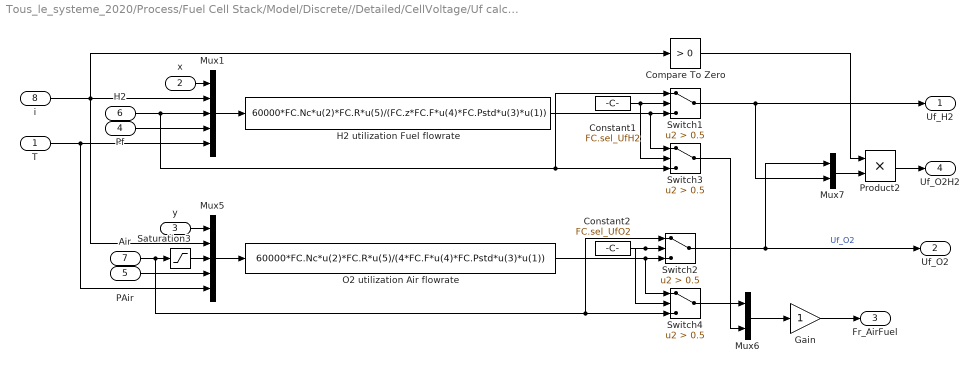
== system Tous_le_systeme_2020/Process/Fuel Cell Stack/Model/Discrete//Detailed/CellVoltage/Uf calculator ==
  T : Inport
  x : Inport  Port=2
  y : Inport  Port=3
  Pf : Inport  Port=4
  PAir : Inport  Port=5
  H2 : Inport  Port=6
  Air : Inport  Port=7
  i : Inport  Port=8
  Compare To Zero : simulink/Logic and Bit Operations/Compare To Zero  relop=>  OutDataTypeStr=uint8
  Constant1 : Constant  Value=FC.sel_UfH2
  Constant2 : Constant  Value=FC.sel_UfO2
  Gain : Gain
  H2 utilization Fuel flowrate : Fcn  Expr=60000*FC.Nc*u(2)*FC.R*u(5)/(FC.z*FC.F*u(4)*FC.Pstd*u(3)*u(1))
  Mux1 : Mux  Inputs=5
  Mux5 : Mux  Inputs=5
  Mux6 : Mux  Inputs=2
  Mux7 : Mux  Inputs=2
  O2 utilization Air flowrate : Fcn  Expr=60000*FC.Nc*u(2)*FC.R*u(5)/(4*FC.F*u(4)*FC.Pstd*u(3)*u(1))
  Product2 : Product  RndMeth=Zero
  Saturation3 : Saturate  UpperLimit=inf  LowerLimit=FC.AirFr_Max*0.01
  Switch{1..4} (4 alike) : Switch  Criteria=u2 > Threshold  Threshold=0.5
  Uf_H2 : Outport  VectorParamsAs1DForOutWhenUnconnected=off
  Uf_O2 : Outport  Port=2  VectorParamsAs1DForOutWhenUnconnected=off
  Fr_AirFuel : Outport  Port=3  VectorParamsAs1DForOutWhenUnconnected=off
  Uf_O2H2 : Outport  Port=4  VectorParamsAs1DForOutWhenUnconnected=off
  wires:
  Compare To Zero/1 -> Product2/1
  Product2/1 -> Uf_O2H2/1
  Mux7/1 -> Product2/2
  Mux1/1 -> H2 utilization Fuel flowrate/1
  Mux5/1 -> O2 utilization Air flowrate/1
  x/1 -> Mux1/1
  H2/1 -> Switch3/3, Switch1/1, Mux1/3
  y/1 -> Mux5/1
  Air/1 -> Switch4/3, Switch2/1, Saturation3/1
  i/1 -> Mux5/2, Mux1/2, Compare To Zero/1
  H2 utilization Fuel flowrate/1 -> Switch1/3, Switch3/1
  Constant1/1 -> Switch1/2, Switch3/2
  Constant2/1 -> Switch2/2, Switch4/2
  O2 utilization Air flowrate/1 -> Switch2/3, Switch4/1
  T/1 -> Mux5/5, Mux1/5
  Pf/1 -> Mux1/4
  PAir/1 -> Mux5/4
  Mux6/1 -> Gain/1
  Switch3/1 -> Mux6/2
  Switch4/1 -> Mux6/1
  Gain/1 -> Fr_AirFuel/1
  Switch2/1 -> Uf_O2/1, Mux7/1  "Uf_O2"
  Saturation3/1 -> Mux5/3
  Switch1/1 -> Uf_H2/1, Mux7/2

== matlab function Tous_le_systeme_2020/ML Model/MATLAB Function2 ==
  data: T input; Vmpp output; Pfuel input; Pair input; Vfuel input; Vair input
function Vmpp = fcn(T, Pfuel, Pair, Vfuel, Vair)

    Vmpp = 0.0; % Predefine output as double to satisfy Simulink
    Vmpp = load_pytorch_model(T, Pfuel, Pair, Vfuel, Vair);
end

== matlab function Tous_le_systeme_2020/ML Model/MATLAB Function1 ==
  data: T input; vmpp output; Pfuel input; Pair input; Vfuel input; Vair input
function vmpp = fcn(T, Pfuel, Pair, Vfuel, Vair)
    vmpp = predict_vmpp(T, Pfuel, Pair, Vfuel, Vair);
end
